simulink model "sei"  (Simulink 6.2)
settings: Solver=ode45  StartTime=0.0  StopTime=10.0  RelTol=1e-3
libraries: dsparch4 x287, cdsEpicsOut x108, cdsEpicsIn x18, cdsRms x18, Matrix8x x15, cdsSwitch1 x12, cdsProduct x9, Matrix88 x9, cdsSwitch x6, cdsSubtract8 x3, cdsRampSwitch x3, cdsSWD1 x3
(part 3 of 6)

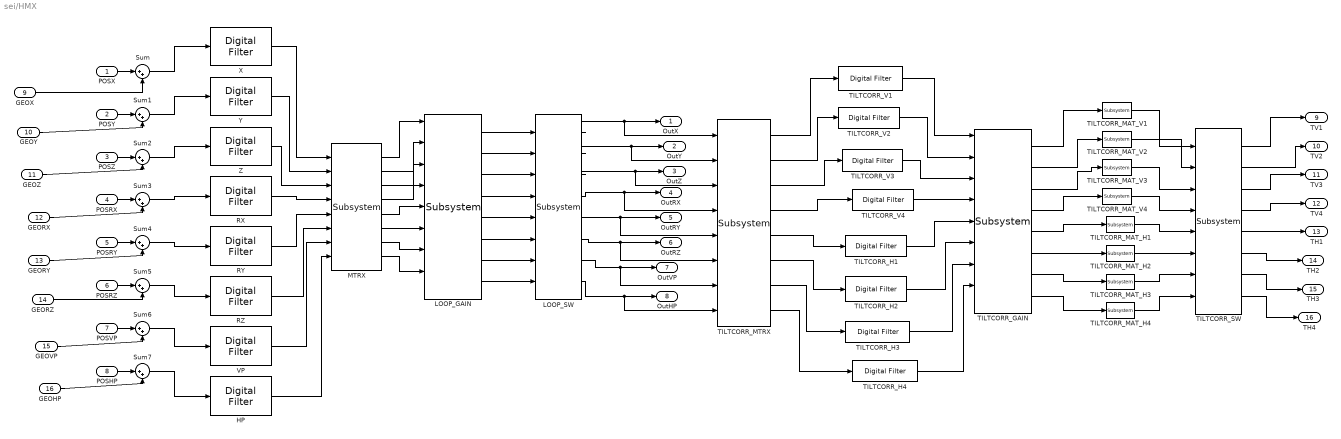
== system sei/HMX ==
  POSX : Inport  Port=1  LatchInput=off
  POSY : Inport  Port=2  LatchInput=off
  POSZ : Inport  Port=3  LatchInput=off
  POSRX : Inport  Port=4  LatchInput=off
  POSRY : Inport  Port=5  LatchInput=off
  POSRZ : Inport  Port=6  LatchInput=off
  POSVP : Inport  Port=7  LatchInput=off
  POSHP : Inport  Port=8  LatchInput=off
  GEOX : Inport  Port=9  LatchInput=off
  GEOY : Inport  Port=10  LatchInput=off
  GEOZ : Inport  Port=11  LatchInput=off
  GEORX : Inport  Port=12  LatchInput=off
  GEORY : Inport  Port=13  LatchInput=off
  GEORZ : Inport  Port=14  LatchInput=off
  GEOVP : Inport  Port=15  LatchInput=off
  GEOHP : Inport  Port=16  LatchInput=off
  HP : dsparch4/Digital Filter  DialogController=dspDDGCreate  DialogControllerArgs=DataTag93  TypePopup=IIR (poles & zeros)  IIRFiltStruct=Direct form II transposed  AllPoleFiltStruct=Direct form  FIRFiltStruct=Direct form  CoeffSource=Specify via dialog  NumCoeffs=[1 2]  DenCoeffs=[1 0.1]  BiQuadCoeffs=[1 0.3 0.4 1 0.1 0.2]  LatticeCoeffs=[0.2 0.4]  denIgnore=on  FiltPerSampPopup=One filter per frame  IC=0  ICnum=0  ICden=0  roundingMode=Floor  overflowMode=off  ScaleValues=1  scaleValueFracLength=14  stageInFracLength=15  stageOutFracLength=15
  LOOP_GAIN : cdsProduct/Subsystem
      settings: AttributesFormatString=%<ReferenceBlock>
  LOOP_SW : cdsSwitch1/Subsystem
      settings: AttributesFormatString=%<ReferenceBlock>
  MTRX : Matrix8x/Subsystem
  RX : dsparch4/Digital Filter  DialogController=dspDDGCreate  DialogControllerArgs=DataTag94  TypePopup=IIR (poles & zeros)  IIRFiltStruct=Direct form II transposed  AllPoleFiltStruct=Direct form  FIRFiltStruct=Direct form  CoeffSource=Specify via dialog  NumCoeffs=[1 2]  DenCoeffs=[1 0.1]  BiQuadCoeffs=[1 0.3 0.4 1 0.1 0.2]  LatticeCoeffs=[0.2 0.4]  denIgnore=on  FiltPerSampPopup=One filter per frame  IC=0  ICnum=0  ICden=0  roundingMode=Floor  overflowMode=off  ScaleValues=1  scaleValueFracLength=14  stageInFracLength=15  stageOutFracLength=15
  RY : dsparch4/Digital Filter  DialogController=dspDDGCreate  DialogControllerArgs=DataTag95  TypePopup=IIR (poles & zeros)  IIRFiltStruct=Direct form II transposed  AllPoleFiltStruct=Direct form  FIRFiltStruct=Direct form  CoeffSource=Specify via dialog  NumCoeffs=[1 2]  DenCoeffs=[1 0.1]  BiQuadCoeffs=[1 0.3 0.4 1 0.1 0.2]  LatticeCoeffs=[0.2 0.4]  denIgnore=on  FiltPerSampPopup=One filter per frame  IC=0  ICnum=0  ICden=0  roundingMode=Floor  overflowMode=off  ScaleValues=1  scaleValueFracLength=14  stageInFracLength=15  stageOutFracLength=15
  RZ : dsparch4/Digital Filter  DialogController=dspDDGCreate  DialogControllerArgs=DataTag96  TypePopup=IIR (poles & zeros)  IIRFiltStruct=Direct form II transposed  AllPoleFiltStruct=Direct form  FIRFiltStruct=Direct form  CoeffSource=Specify via dialog  NumCoeffs=[1 2]  DenCoeffs=[1 0.1]  BiQuadCoeffs=[1 0.3 0.4 1 0.1 0.2]  LatticeCoeffs=[0.2 0.4]  denIgnore=on  FiltPerSampPopup=One filter per frame  IC=0  ICnum=0  ICden=0  roundingMode=Floor  overflowMode=off  ScaleValues=1  scaleValueFracLength=14  stageInFracLength=15  stageOutFracLength=15
  Sum{,1..7} (8 alike) : Sum  Inputs=|++
  TILTCORR_GAIN : cdsProduct/Subsystem
      settings: AttributesFormatString=%<ReferenceBlock>
  TILTCORR_H1 : dsparch4/Digital Filter  DialogController=dspDDGCreate  DialogControllerArgs=DataTag97  TypePopup=IIR (poles & zeros)  IIRFiltStruct=Direct form II transposed  AllPoleFiltStruct=Direct form  FIRFiltStruct=Direct form  CoeffSource=Specify via dialog  NumCoeffs=[1 2]  DenCoeffs=[1 0.1]  BiQuadCoeffs=[1 0.3 0.4 1 0.1 0.2]  LatticeCoeffs=[0.2 0.4]  denIgnore=on  FiltPerSampPopup=One filter per frame  IC=0  ICnum=0  ICden=0  roundingMode=Floor  overflowMode=off  ScaleValues=1  scaleValueFracLength=14  stageInFracLength=15  stageOutFracLength=15
  TILTCORR_H2 : dsparch4/Digital Filter  DialogController=dspDDGCreate  DialogControllerArgs=DataTag98  TypePopup=IIR (poles & zeros)  IIRFiltStruct=Direct form II transposed  AllPoleFiltStruct=Direct form  FIRFiltStruct=Direct form  CoeffSource=Specify via dialog  NumCoeffs=[1 2]  DenCoeffs=[1 0.1]  BiQuadCoeffs=[1 0.3 0.4 1 0.1 0.2]  LatticeCoeffs=[0.2 0.4]  denIgnore=on  FiltPerSampPopup=One filter per frame  IC=0  ICnum=0  ICden=0  roundingMode=Floor  overflowMode=off  ScaleValues=1  scaleValueFracLength=14  stageInFracLength=15  stageOutFracLength=15
  TILTCORR_H3 : dsparch4/Digital Filter  DialogController=dspDDGCreate  DialogControllerArgs=DataTag99  TypePopup=IIR (poles & zeros)  IIRFiltStruct=Direct form II transposed  AllPoleFiltStruct=Direct form  FIRFiltStruct=Direct form  CoeffSource=Specify via dialog  NumCoeffs=[1 2]  DenCoeffs=[1 0.1]  BiQuadCoeffs=[1 0.3 0.4 1 0.1 0.2]  LatticeCoeffs=[0.2 0.4]  denIgnore=on  FiltPerSampPopup=One filter per frame  IC=0  ICnum=0  ICden=0  roundingMode=Floor  overflowMode=off  ScaleValues=1  scaleValueFracLength=14  stageInFracLength=15  stageOutFracLength=15
  TILTCORR_H4 : dsparch4/Digital Filter  DialogController=dspDDGCreate  DialogControllerArgs=DataTag100  TypePopup=IIR (poles & zeros)  IIRFiltStruct=Direct form II transposed  AllPoleFiltStruct=Direct form  FIRFiltStruct=Direct form  CoeffSource=Specify via dialog  NumCoeffs=[1 2]  DenCoeffs=[1 0.1]  BiQuadCoeffs=[1 0.3 0.4 1 0.1 0.2]  LatticeCoeffs=[0.2 0.4]  denIgnore=on  FiltPerSampPopup=One filter per frame  IC=0  ICnum=0  ICden=0  roundingMode=Floor  overflowMode=off  ScaleValues=1  scaleValueFracLength=14  stageInFracLength=15  stageOutFracLength=15
  TILTCORR_MAT_H{1..4} (4 alike) : cdsEpicsOut/Subsystem
  TILTCORR_MAT_V{1..4} (4 alike) : cdsEpicsOut/Subsystem
  TILTCORR_MTRX : Matrix8x/Subsystem
  TILTCORR_SW : cdsSwitch1/Subsystem
      settings: AttributesFormatString=%<ReferenceBlock>
  TILTCORR_V1 : dsparch4/Digital Filter  DialogController=dspDDGCreate  DialogControllerArgs=DataTag101  TypePopup=IIR (poles & zeros)  IIRFiltStruct=Direct form II transposed  AllPoleFiltStruct=Direct form  FIRFiltStruct=Direct form  CoeffSource=Specify via dialog  NumCoeffs=[1 2]  DenCoeffs=[1 0.1]  BiQuadCoeffs=[1 0.3 0.4 1 0.1 0.2]  LatticeCoeffs=[0.2 0.4]  denIgnore=on  FiltPerSampPopup=One filter per frame  IC=0  ICnum=0  ICden=0  roundingMode=Floor  overflowMode=off  ScaleValues=1  scaleValueFracLength=14  stageInFracLength=15  stageOutFracLength=15
  TILTCORR_V2 : dsparch4/Digital Filter  DialogController=dspDDGCreate  DialogControllerArgs=DataTag102  TypePopup=IIR (poles & zeros)  IIRFiltStruct=Direct form II transposed  AllPoleFiltStruct=Direct form  FIRFiltStruct=Direct form  CoeffSource=Specify via dialog  NumCoeffs=[1 2]  DenCoeffs=[1 0.1]  BiQuadCoeffs=[1 0.3 0.4 1 0.1 0.2]  LatticeCoeffs=[0.2 0.4]  denIgnore=on  FiltPerSampPopup=One filter per frame  IC=0  ICnum=0  ICden=0  roundingMode=Floor  overflowMode=off  ScaleValues=1  scaleValueFracLength=14  stageInFracLength=15  stageOutFracLength=15
  TILTCORR_V3 : dsparch4/Digital Filter  DialogController=dspDDGCreate  DialogControllerArgs=DataTag103  TypePopup=IIR (poles & zeros)  IIRFiltStruct=Direct form II transposed  AllPoleFiltStruct=Direct form  FIRFiltStruct=Direct form  CoeffSource=Specify via dialog  NumCoeffs=[1 2]  DenCoeffs=[1 0.1]  BiQuadCoeffs=[1 0.3 0.4 1 0.1 0.2]  LatticeCoeffs=[0.2 0.4]  denIgnore=on  FiltPerSampPopup=One filter per frame  IC=0  ICnum=0  ICden=0  roundingMode=Floor  overflowMode=off  ScaleValues=1  scaleValueFracLength=14  stageInFracLength=15  stageOutFracLength=15
  TILTCORR_V4 : dsparch4/Digital Filter  DialogController=dspDDGCreate  DialogControllerArgs=DataTag104  TypePopup=IIR (poles & zeros)  IIRFiltStruct=Direct form II transposed  AllPoleFiltStruct=Direct form  FIRFiltStruct=Direct form  CoeffSource=Specify via dialog  NumCoeffs=[1 2]  DenCoeffs=[1 0.1]  BiQuadCoeffs=[1 0.3 0.4 1 0.1 0.2]  LatticeCoeffs=[0.2 0.4]  denIgnore=on  FiltPerSampPopup=One filter per frame  IC=0  ICnum=0  ICden=0  roundingMode=Floor  overflowMode=off  ScaleValues=1  scaleValueFracLength=14  stageInFracLength=15  stageOutFracLength=15
  VP : dsparch4/Digital Filter  DialogController=dspDDGCreate  DialogControllerArgs=DataTag105  TypePopup=IIR (poles & zeros)  IIRFiltStruct=Direct form II transposed  AllPoleFiltStruct=Direct form  FIRFiltStruct=Direct form  CoeffSource=Specify via dialog  NumCoeffs=[1 2]  DenCoeffs=[1 0.1]  BiQuadCoeffs=[1 0.3 0.4 1 0.1 0.2]  LatticeCoeffs=[0.2 0.4]  denIgnore=on  FiltPerSampPopup=One filter per frame  IC=0  ICnum=0  ICden=0  roundingMode=Floor  overflowMode=off  ScaleValues=1  scaleValueFracLength=14  stageInFracLength=15  stageOutFracLength=15
  X : dsparch4/Digital Filter  DialogController=dspDDGCreate  DialogControllerArgs=DataTag106  TypePopup=IIR (poles & zeros)  IIRFiltStruct=Direct form II transposed  AllPoleFiltStruct=Direct form  FIRFiltStruct=Direct form  CoeffSource=Specify via dialog  NumCoeffs=[1 2]  DenCoeffs=[1 0.1]  BiQuadCoeffs=[1 0.3 0.4 1 0.1 0.2]  LatticeCoeffs=[0.2 0.4]  denIgnore=on  FiltPerSampPopup=One filter per frame  IC=0  ICnum=0  ICden=0  roundingMode=Floor  overflowMode=off  ScaleValues=1  scaleValueFracLength=14  stageInFracLength=15  stageOutFracLength=15
  Y : dsparch4/Digital Filter  DialogController=dspDDGCreate  DialogControllerArgs=DataTag107  TypePopup=IIR (poles & zeros)  IIRFiltStruct=Direct form II transposed  AllPoleFiltStruct=Direct form  FIRFiltStruct=Direct form  CoeffSource=Specify via dialog  NumCoeffs=[1 2]  DenCoeffs=[1 0.1]  BiQuadCoeffs=[1 0.3 0.4 1 0.1 0.2]  LatticeCoeffs=[0.2 0.4]  denIgnore=on  FiltPerSampPopup=One filter per frame  IC=0  ICnum=0  ICden=0  roundingMode=Floor  overflowMode=off  ScaleValues=1  scaleValueFracLength=14  stageInFracLength=15  stageOutFracLength=15
  Z : dsparch4/Digital Filter  DialogController=dspDDGCreate  DialogControllerArgs=DataTag108  TypePopup=IIR (poles & zeros)  IIRFiltStruct=Direct form II transposed  AllPoleFiltStruct=Direct form  FIRFiltStruct=Direct form  CoeffSource=Specify via dialog  NumCoeffs=[1 2]  DenCoeffs=[1 0.1]  BiQuadCoeffs=[1 0.3 0.4 1 0.1 0.2]  LatticeCoeffs=[0.2 0.4]  denIgnore=on  FiltPerSampPopup=One filter per frame  IC=0  ICnum=0  ICden=0  roundingMode=Floor  overflowMode=off  ScaleValues=1  scaleValueFracLength=14  stageInFracLength=15  stageOutFracLength=15
  OutX : Outport
  OutY : Outport  Port=2
  OutZ : Outport  Port=3
  OutRX : Outport  Port=4
  OutRY : Outport  Port=5
  OutRZ : Outport  Port=6
  OutVP : Outport  Port=7
  OutHP : Outport  Port=8
  TV1 : Outport  Port=9
  TV2 : Outport  Port=10
  TV3 : Outport  Port=11
  TV4 : Outport  Port=12
  TH1 : Outport  Port=13
  TH2 : Outport  Port=14
  TH3 : Outport  Port=15
  TH4 : Outport  Port=16
  wires:
  Sum/1 -> X/1
  Sum1/1 -> Y/1
  Sum2/1 -> Z/1
  Sum3/1 -> RX/1
  Sum4/1 -> RY/1
  Sum5/1 -> RZ/1
  Sum6/1 -> VP/1
  Sum7/1 -> HP/1
  X/1 -> MTRX/1
  Y/1 -> MTRX/2
  Z/1 -> MTRX/3
  RX/1 -> MTRX/4
  RY/1 -> MTRX/5
  RZ/1 -> MTRX/6
  VP/1 -> MTRX/7
  HP/1 -> MTRX/8
  POSX/1 -> Sum/1
  GEOX/1 -> Sum/2
  POSY/1 -> Sum1/1
  GEOY/1 -> Sum1/2
  POSZ/1 -> Sum2/1
  GEOZ/1 -> Sum2/2
  POSRX/1 -> Sum3/1
  GEORX/1 -> Sum3/2
  POSRY/1 -> Sum4/1
  GEORY/1 -> Sum4/2
  POSRZ/1 -> Sum5/1
  GEORZ/1 -> Sum5/2
  POSVP/1 -> Sum6/1
  GEOVP/1 -> Sum6/2
  POSHP/1 -> Sum7/1
  GEOHP/1 -> Sum7/2
  LOOP_GAIN/1 -> LOOP_SW/1
  LOOP_GAIN/2 -> LOOP_SW/2
  LOOP_GAIN/3 -> LOOP_SW/3
  LOOP_GAIN/4 -> LOOP_SW/4
  LOOP_GAIN/5 -> LOOP_SW/5
  LOOP_GAIN/6 -> LOOP_SW/6
  LOOP_GAIN/7 -> LOOP_SW/7
  LOOP_GAIN/8 -> LOOP_SW/8
  LOOP_SW/1 -> OutX/1, TILTCORR_MTRX/1
  LOOP_SW/2 -> OutY/1, TILTCORR_MTRX/2
  LOOP_SW/3 -> OutZ/1, TILTCORR_MTRX/3
  LOOP_SW/4 -> OutRX/1, TILTCORR_MTRX/4
  LOOP_SW/5 -> OutRY/1, TILTCORR_MTRX/5
  LOOP_SW/6 -> OutRZ/1, TILTCORR_MTRX/6
  LOOP_SW/7 -> OutVP/1, TILTCORR_MTRX/7
  LOOP_SW/8 -> OutHP/1, TILTCORR_MTRX/8
  MTRX/1 -> LOOP_GAIN/1
  MTRX/2 -> LOOP_GAIN/2
  MTRX/3 -> LOOP_GAIN/3
  MTRX/4 -> LOOP_GAIN/4
  MTRX/5 -> LOOP_GAIN/5
  MTRX/6 -> LOOP_GAIN/6
  MTRX/7 -> LOOP_GAIN/7
  MTRX/8 -> LOOP_GAIN/8
  TILTCORR_MTRX/1 -> TILTCORR_V1/1
  TILTCORR_MTRX/2 -> TILTCORR_V2/1
  TILTCORR_MTRX/3 -> TILTCORR_V3/1
  TILTCORR_MTRX/4 -> TILTCORR_V4/1
  TILTCORR_MTRX/5 -> TILTCORR_H1/1
  TILTCORR_MTRX/6 -> TILTCORR_H2/1
  TILTCORR_MTRX/7 -> TILTCORR_H3/1
  TILTCORR_MTRX/8 -> TILTCORR_H4/1
  TILTCORR_V1/1 -> TILTCORR_GAIN/1
  TILTCORR_V2/1 -> TILTCORR_GAIN/2
  TILTCORR_V3/1 -> TILTCORR_GAIN/3
  TILTCORR_V4/1 -> TILTCORR_GAIN/4
  TILTCORR_H1/1 -> TILTCORR_GAIN/5
  TILTCORR_H2/1 -> TILTCORR_GAIN/6
  TILTCORR_H3/1 -> TILTCORR_GAIN/7
  TILTCORR_H4/1 -> TILTCORR_GAIN/8
  TILTCORR_GAIN/1 -> TILTCORR_MAT_V1/1
  TILTCORR_GAIN/2 -> TILTCORR_MAT_V2/1
  TILTCORR_GAIN/3 -> TILTCORR_MAT_V3/1
  TILTCORR_GAIN/4 -> TILTCORR_MAT_V4/1
  TILTCORR_GAIN/5 -> TILTCORR_MAT_H1/1
  TILTCORR_GAIN/6 -> TILTCORR_MAT_H2/1
  TILTCORR_GAIN/7 -> TILTCORR_MAT_H3/1
  TILTCORR_GAIN/8 -> TILTCORR_MAT_H4/1
  TILTCORR_MAT_V1/1 -> TILTCORR_SW/1
  TILTCORR_MAT_V2/1 -> TILTCORR_SW/2
  TILTCORR_MAT_V3/1 -> TILTCORR_SW/3
  TILTCORR_MAT_V4/1 -> TILTCORR_SW/4
  TILTCORR_MAT_H1/1 -> TILTCORR_SW/5
  TILTCORR_MAT_H2/1 -> TILTCORR_SW/6
  TILTCORR_MAT_H3/1 -> TILTCORR_SW/7
  TILTCORR_MAT_H4/1 -> TILTCORR_SW/8
  TILTCORR_SW/1 -> TV1/1
  TILTCORR_SW/2 -> TV2/1
  TILTCORR_SW/3 -> TV3/1
  TILTCORR_SW/4 -> TV4/1
  TILTCORR_SW/5 -> TH1/1
  TILTCORR_SW/6 -> TH2/1
  TILTCORR_SW/7 -> TH3/1
  TILTCORR_SW/8 -> TH4/1

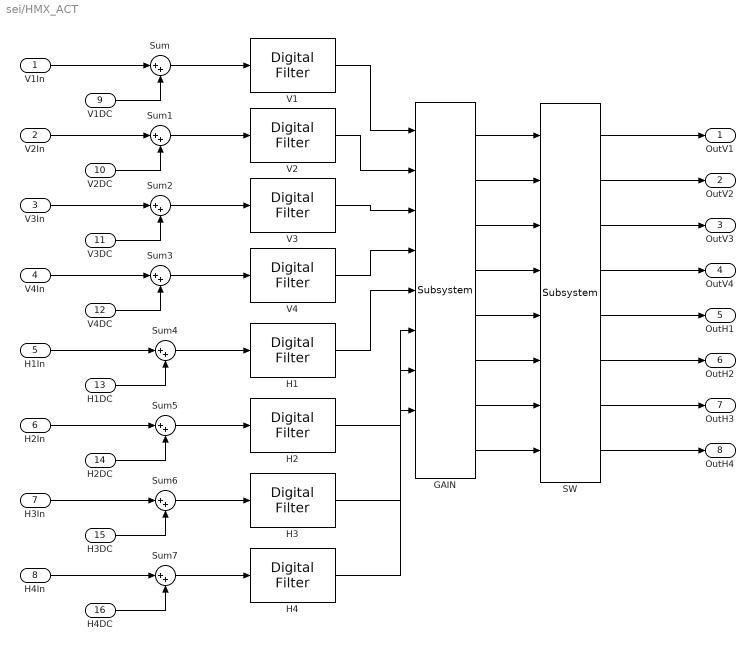
== system sei/HMX_ACT ==
  V1In : Inport  Port=1  LatchInput=off
  V2In : Inport  Port=2  LatchInput=off
  V3In : Inport  Port=3  LatchInput=off
  V4In : Inport  Port=4  LatchInput=off
  H1In : Inport  Port=5  LatchInput=off
  H2In : Inport  Port=6  LatchInput=off
  H3In : Inport  Port=7  LatchInput=off
  H4In : Inport  Port=8  LatchInput=off
  V1DC : Inport  Port=9  LatchInput=off
  V2DC : Inport  Port=10  LatchInput=off
  V3DC : Inport  Port=11  LatchInput=off
  V4DC : Inport  Port=12  LatchInput=off
  H1DC : Inport  Port=13  LatchInput=off
  H2DC : Inport  Port=14  LatchInput=off
  H3DC : Inport  Port=15  LatchInput=off
  H4DC : Inport  Port=16  LatchInput=off
  GAIN : cdsProduct/Subsystem
  H1 : dsparch4/Digital Filter  DialogController=dspDDGCreate  DialogControllerArgs=DataTag109  TypePopup=IIR (poles & zeros)  IIRFiltStruct=Direct form II transposed  AllPoleFiltStruct=Direct form  FIRFiltStruct=Direct form  CoeffSource=Specify via dialog  NumCoeffs=[1 2]  DenCoeffs=[1 0.1]  BiQuadCoeffs=[1 0.3 0.4 1 0.1 0.2]  LatticeCoeffs=[0.2 0.4]  denIgnore=on  FiltPerSampPopup=One filter per frame  IC=0  ICnum=0  ICden=0  roundingMode=Floor  overflowMode=off  ScaleValues=1  scaleValueFracLength=14  stageInFracLength=15  stageOutFracLength=15
  H2 : dsparch4/Digital Filter  DialogController=dspDDGCreate  DialogControllerArgs=DataTag110  TypePopup=IIR (poles & zeros)  IIRFiltStruct=Direct form II transposed  AllPoleFiltStruct=Direct form  FIRFiltStruct=Direct form  CoeffSource=Specify via dialog  NumCoeffs=[1 2]  DenCoeffs=[1 0.1]  BiQuadCoeffs=[1 0.3 0.4 1 0.1 0.2]  LatticeCoeffs=[0.2 0.4]  denIgnore=on  FiltPerSampPopup=One filter per frame  IC=0  ICnum=0  ICden=0  roundingMode=Floor  overflowMode=off  ScaleValues=1  scaleValueFracLength=14  stageInFracLength=15  stageOutFracLength=15
  H3 : dsparch4/Digital Filter  DialogController=dspDDGCreate  DialogControllerArgs=DataTag111  TypePopup=IIR (poles & zeros)  IIRFiltStruct=Direct form II transposed  AllPoleFiltStruct=Direct form  FIRFiltStruct=Direct form  CoeffSource=Specify via dialog  NumCoeffs=[1 2]  DenCoeffs=[1 0.1]  BiQuadCoeffs=[1 0.3 0.4 1 0.1 0.2]  LatticeCoeffs=[0.2 0.4]  denIgnore=on  FiltPerSampPopup=One filter per frame  IC=0  ICnum=0  ICden=0  roundingMode=Floor  overflowMode=off  ScaleValues=1  scaleValueFracLength=14  stageInFracLength=15  stageOutFracLength=15
  H4 : dsparch4/Digital Filter  DialogController=dspDDGCreate  DialogControllerArgs=DataTag112  TypePopup=IIR (poles & zeros)  IIRFiltStruct=Direct form II transposed  AllPoleFiltStruct=Direct form  FIRFiltStruct=Direct form  CoeffSource=Specify via dialog  NumCoeffs=[1 2]  DenCoeffs=[1 0.1]  BiQuadCoeffs=[1 0.3 0.4 1 0.1 0.2]  LatticeCoeffs=[0.2 0.4]  denIgnore=on  FiltPerSampPopup=One filter per frame  IC=0  ICnum=0  ICden=0  roundingMode=Floor  overflowMode=off  ScaleValues=1  scaleValueFracLength=14  stageInFracLength=15  stageOutFracLength=15
  SW : cdsSwitch1/Subsystem
  Sum{,1..7} (8 alike) : Sum  Inputs=|++
  V1 : dsparch4/Digital Filter  DialogController=dspDDGCreate  DialogControllerArgs=DataTag113  TypePopup=IIR (poles & zeros)  IIRFiltStruct=Direct form II transposed  AllPoleFiltStruct=Direct form  FIRFiltStruct=Direct form  CoeffSource=Specify via dialog  NumCoeffs=[1 2]  DenCoeffs=[1 0.1]  BiQuadCoeffs=[1 0.3 0.4 1 0.1 0.2]  LatticeCoeffs=[0.2 0.4]  denIgnore=on  FiltPerSampPopup=One filter per frame  IC=0  ICnum=0  ICden=0  roundingMode=Floor  overflowMode=off  ScaleValues=1  scaleValueFracLength=14  stageInFracLength=15  stageOutFracLength=15
  V2 : dsparch4/Digital Filter  DialogController=dspDDGCreate  DialogControllerArgs=DataTag114  TypePopup=IIR (poles & zeros)  IIRFiltStruct=Direct form II transposed  AllPoleFiltStruct=Direct form  FIRFiltStruct=Direct form  CoeffSource=Specify via dialog  NumCoeffs=[1 2]  DenCoeffs=[1 0.1]  BiQuadCoeffs=[1 0.3 0.4 1 0.1 0.2]  LatticeCoeffs=[0.2 0.4]  denIgnore=on  FiltPerSampPopup=One filter per frame  IC=0  ICnum=0  ICden=0  roundingMode=Floor  overflowMode=off  ScaleValues=1  scaleValueFracLength=14  stageInFracLength=15  stageOutFracLength=15
  V3 : dsparch4/Digital Filter  DialogController=dspDDGCreate  DialogControllerArgs=DataTag115  TypePopup=IIR (poles & zeros)  IIRFiltStruct=Direct form II transposed  AllPoleFiltStruct=Direct form  FIRFiltStruct=Direct form  CoeffSource=Specify via dialog  NumCoeffs=[1 2]  DenCoeffs=[1 0.1]  BiQuadCoeffs=[1 0.3 0.4 1 0.1 0.2]  LatticeCoeffs=[0.2 0.4]  denIgnore=on  FiltPerSampPopup=One filter per frame  IC=0  ICnum=0  ICden=0  roundingMode=Floor  overflowMode=off  ScaleValues=1  scaleValueFracLength=14  stageInFracLength=15  stageOutFracLength=15
  V4 : dsparch4/Digital Filter  DialogController=dspDDGCreate  DialogControllerArgs=DataTag116  TypePopup=IIR (poles & zeros)  IIRFiltStruct=Direct form II transposed  AllPoleFiltStruct=Direct form  FIRFiltStruct=Direct form  CoeffSource=Specify via dialog  NumCoeffs=[1 2]  DenCoeffs=[1 0.1]  BiQuadCoeffs=[1 0.3 0.4 1 0.1 0.2]  LatticeCoeffs=[0.2 0.4]  denIgnore=on  FiltPerSampPopup=One filter per frame  IC=0  ICnum=0  ICden=0  roundingMode=Floor  overflowMode=off  ScaleValues=1  scaleValueFracLength=14  stageInFracLength=15  stageOutFracLength=15
  OutV1 : Outport
  OutV2 : Outport  Port=2
  OutV3 : Outport  Port=3
  OutV4 : Outport  Port=4
  OutH1 : Outport  Port=5
  OutH2 : Outport  Port=6
  OutH3 : Outport  Port=7
  OutH4 : Outport  Port=8
  wires:
  GAIN/1 -> SW/1
  GAIN/2 -> SW/2
  GAIN/3 -> SW/3
  GAIN/4 -> SW/4
  GAIN/5 -> SW/5
  GAIN/6 -> SW/6
  GAIN/7 -> SW/7
  GAIN/8 -> SW/8
  V1DC/1 -> Sum/2
  V2DC/1 -> Sum1/2
  V3DC/1 -> Sum2/2
  V4DC/1 -> Sum3/2
  H1DC/1 -> Sum4/2
  H2DC/1 -> Sum5/2
  H3DC/1 -> Sum6/2
  H4DC/1 -> Sum7/2
  Sum4/1 -> H1/1
  Sum5/1 -> H2/1
  Sum6/1 -> H3/1
  Sum7/1 -> H4/1
  Sum3/1 -> V4/1
  Sum2/1 -> V3/1
  Sum1/1 -> V2/1
  Sum/1 -> V1/1
  V1In/1 -> Sum/1
  V2In/1 -> Sum1/1
  V3In/1 -> Sum2/1
  V4In/1 -> Sum3/1
  H1In/1 -> Sum4/1
  H2In/1 -> Sum5/1
  H3In/1 -> Sum6/1
  H4In/1 -> Sum7/1
  V1/1 -> GAIN/1
  V2/1 -> GAIN/2
  V3/1 -> GAIN/3
  V4/1 -> GAIN/4
  H1/1 -> GAIN/5
  H2/1 -> GAIN/6
  H3/1 -> GAIN/7
  H4/1 -> GAIN/8
  SW/1 -> OutV1/1
  SW/2 -> OutV2/1
  SW/3 -> OutV3/1
  SW/4 -> OutV4/1
  SW/5 -> OutH1/1
  SW/6 -> OutH2/1
  SW/7 -> OutH3/1
  SW/8 -> OutH4/1

== system sei/HMX_DC_BIAS ==
  {1..6} (6 alike) : cdsEpicsIn/Subsystem
  MTRX : Matrix8x/Subsystem
  SW : cdsSwitch1/Subsystem
  V1 : Outport
  V2 : Outport  Port=2
  V3 : Outport  Port=3
  V4 : Outport  Port=4
  H1 : Outport  Port=5
  H2 : Outport  Port=6
  H3 : Outport  Port=7
  H4 : Outport  Port=8
  wires:
  1/1 -> MTRX/1
  2/1 -> MTRX/2
  3/1 -> MTRX/3
  4/1 -> MTRX/4
  5/1 -> MTRX/5
  6/1 -> MTRX/6
  MTRX/1 -> SW/1
  MTRX/2 -> SW/2
  MTRX/3 -> SW/3
  MTRX/4 -> SW/4
  MTRX/5 -> SW/5
  MTRX/6 -> SW/6
  MTRX/7 -> SW/7
  MTRX/8 -> SW/8
  SW/1 -> V1/1
  SW/2 -> V2/1
  SW/3 -> V3/1
  SW/4 -> V4/1
  SW/5 -> H1/1
  SW/6 -> H2/1
  SW/7 -> H3/1
  SW/8 -> H4/1

== system sei/HMX_FIR ==
  X1 : Inport  Port=1  LatchInput=off
  Y1 : Inport  Port=2  LatchInput=off
  X2 : Inport  Port=3  LatchInput=off
  Y2 : Inport  Port=4  LatchInput=off
  MTRX : Matrix88/Subsystem
  X_OUT : dsparch4/Digital Filter  DialogController=dspDDGCreate  DialogControllerArgs=DataTag117  TypePopup=IIR (poles & zeros)  IIRFiltStruct=Direct form II transposed  AllPoleFiltStruct=Direct form  FIRFiltStruct=Direct form  CoeffSource=Specify via dialog  NumCoeffs=[1 2]  DenCoeffs=[1 0.1]  BiQuadCoeffs=[1 0.3 0.4 1 0.1 0.2]  LatticeCoeffs=[0.2 0.4]  denIgnore=on  FiltPerSampPopup=One filter per frame  IC=0  ICnum=0  ICden=0  roundingMode=Floor  overflowMode=off  ScaleValues=1  scaleValueFracLength=14  stageInFracLength=15  stageOutFracLength=15
  Y_OUT : dsparch4/Digital Filter  DialogController=dspDDGCreate  DialogControllerArgs=DataTag118  TypePopup=IIR (poles & zeros)  IIRFiltStruct=Direct form II transposed  AllPoleFiltStruct=Direct form  FIRFiltStruct=Direct form  CoeffSource=Specify via dialog  NumCoeffs=[1 2]  DenCoeffs=[1 0.1]  BiQuadCoeffs=[1 0.3 0.4 1 0.1 0.2]  LatticeCoeffs=[0.2 0.4]  denIgnore=on  FiltPerSampPopup=One filter per frame  IC=0  ICnum=0  ICden=0  roundingMode=Floor  overflowMode=off  ScaleValues=1  scaleValueFracLength=14  stageInFracLength=15  stageOutFracLength=15
  X : Outport
  Y : Outport  Port=2
  wires:
  MTRX/1 -> X_OUT/1
  MTRX/2 -> Y_OUT/1
  X1/1 -> MTRX/1
  X_OUT/1 -> X/1
  Y1/1 -> MTRX/2
  X2/1 -> MTRX/3
  Y2/1 -> MTRX/4
  Y_OUT/1 -> Y/1

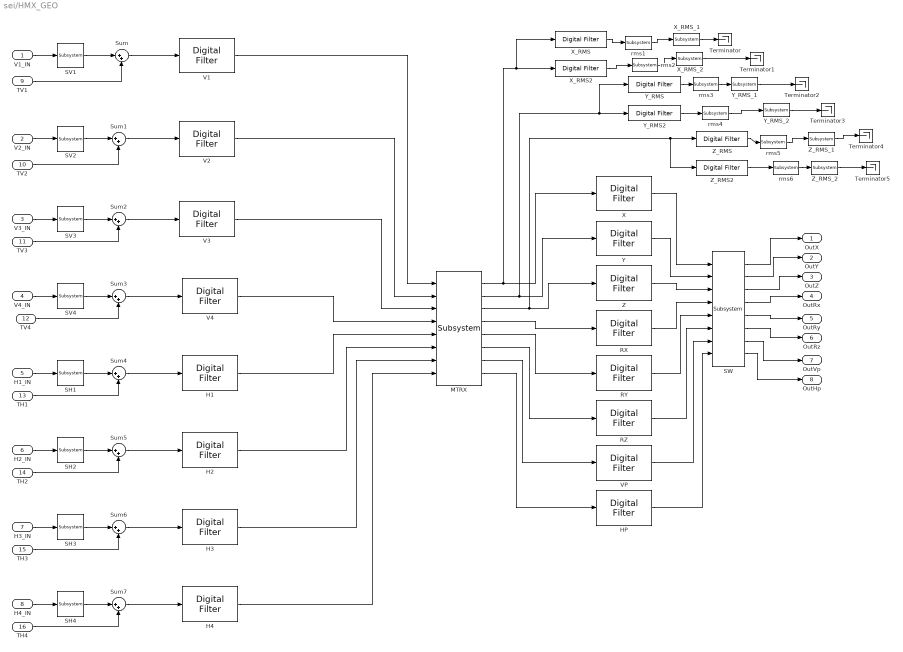
== system sei/HMX_GEO ==
  V1_IN : Inport  Port=1  LatchInput=off
  V2_IN : Inport  Port=2  LatchInput=off
  V3_IN : Inport  Port=3  LatchInput=off
  V4_IN : Inport  Port=4  LatchInput=off
  H1_IN : Inport  Port=5  LatchInput=off
  H2_IN : Inport  Port=6  LatchInput=off
  H3_IN : Inport  Port=7  LatchInput=off
  H4_IN : Inport  Port=8  LatchInput=off
  TV1 : Inport  Port=9  LatchInput=off
  TV2 : Inport  Port=10  LatchInput=off
  TV3 : Inport  Port=11  LatchInput=off
  TV4 : Inport  Port=12  LatchInput=off
  TH1 : Inport  Port=13  LatchInput=off
  TH2 : Inport  Port=14  LatchInput=off
  TH3 : Inport  Port=15  LatchInput=off
  TH4 : Inport  Port=16  LatchInput=off
  H1 : dsparch4/Digital Filter  DialogController=dspDDGCreate  DialogControllerArgs=DataTag119  TypePopup=IIR (poles & zeros)  IIRFiltStruct=Direct form II transposed  AllPoleFiltStruct=Direct form  FIRFiltStruct=Direct form  CoeffSource=Specify via dialog  NumCoeffs=[1 2]  DenCoeffs=[1 0.1]  BiQuadCoeffs=[1 0.3 0.4 1 0.1 0.2]  LatticeCoeffs=[0.2 0.4]  denIgnore=on  FiltPerSampPopup=One filter per frame  IC=0  ICnum=0  ICden=0  roundingMode=Floor  overflowMode=off  ScaleValues=1  scaleValueFracLength=14  stageInFracLength=15  stageOutFracLength=15
  H2 : dsparch4/Digital Filter  DialogController=dspDDGCreate  DialogControllerArgs=DataTag120  TypePopup=IIR (poles & zeros)  IIRFiltStruct=Direct form II transposed  AllPoleFiltStruct=Direct form  FIRFiltStruct=Direct form  CoeffSource=Specify via dialog  NumCoeffs=[1 2]  DenCoeffs=[1 0.1]  BiQuadCoeffs=[1 0.3 0.4 1 0.1 0.2]  LatticeCoeffs=[0.2 0.4]  denIgnore=on  FiltPerSampPopup=One filter per frame  IC=0  ICnum=0  ICden=0  roundingMode=Floor  overflowMode=off  ScaleValues=1  scaleValueFracLength=14  stageInFracLength=15  stageOutFracLength=15
  H3 : dsparch4/Digital Filter  DialogController=dspDDGCreate  DialogControllerArgs=DataTag121  TypePopup=IIR (poles & zeros)  IIRFiltStruct=Direct form II transposed  AllPoleFiltStruct=Direct form  FIRFiltStruct=Direct form  CoeffSource=Specify via dialog  NumCoeffs=[1 2]  DenCoeffs=[1 0.1]  BiQuadCoeffs=[1 0.3 0.4 1 0.1 0.2]  LatticeCoeffs=[0.2 0.4]  denIgnore=on  FiltPerSampPopup=One filter per frame  IC=0  ICnum=0  ICden=0  roundingMode=Floor  overflowMode=off  ScaleValues=1  scaleValueFracLength=14  stageInFracLength=15  stageOutFracLength=15
  H4 : dsparch4/Digital Filter  DialogController=dspDDGCreate  DialogControllerArgs=DataTag122  TypePopup=IIR (poles & zeros)  IIRFiltStruct=Direct form II transposed  AllPoleFiltStruct=Direct form  FIRFiltStruct=Direct form  CoeffSource=Specify via dialog  NumCoeffs=[1 2]  DenCoeffs=[1 0.1]  BiQuadCoeffs=[1 0.3 0.4 1 0.1 0.2]  LatticeCoeffs=[0.2 0.4]  denIgnore=on  FiltPerSampPopup=One filter per frame  IC=0  ICnum=0  ICden=0  roundingMode=Floor  overflowMode=off  ScaleValues=1  scaleValueFracLength=14  stageInFracLength=15  stageOutFracLength=15
  HP : dsparch4/Digital Filter  DialogController=dspDDGCreate  DialogControllerArgs=DataTag123  TypePopup=IIR (poles & zeros)  IIRFiltStruct=Direct form II transposed  AllPoleFiltStruct=Direct form  FIRFiltStruct=Direct form  CoeffSource=Specify via dialog  NumCoeffs=[1 2]  DenCoeffs=[1 0.1]  BiQuadCoeffs=[1 0.3 0.4 1 0.1 0.2]  LatticeCoeffs=[0.2 0.4]  denIgnore=on  FiltPerSampPopup=One filter per frame  IC=0  ICnum=0  ICden=0  roundingMode=Floor  overflowMode=off  ScaleValues=1  scaleValueFracLength=14  stageInFracLength=15  stageOutFracLength=15
  MTRX : Matrix8x/Subsystem
  RX : dsparch4/Digital Filter  DialogController=dspDDGCreate  DialogControllerArgs=DataTag124  TypePopup=IIR (poles & zeros)  IIRFiltStruct=Direct form II transposed  AllPoleFiltStruct=Direct form  FIRFiltStruct=Direct form  CoeffSource=Specify via dialog  NumCoeffs=[1 2]  DenCoeffs=[1 0.1]  BiQuadCoeffs=[1 0.3 0.4 1 0.1 0.2]  LatticeCoeffs=[0.2 0.4]  denIgnore=on  FiltPerSampPopup=One filter per frame  IC=0  ICnum=0  ICden=0  roundingMode=Floor  overflowMode=off  ScaleValues=1  scaleValueFracLength=14  stageInFracLength=15  stageOutFracLength=15
  RY : dsparch4/Digital Filter  DialogController=dspDDGCreate  DialogControllerArgs=DataTag125  TypePopup=IIR (poles & zeros)  IIRFiltStruct=Direct form II transposed  AllPoleFiltStruct=Direct form  FIRFiltStruct=Direct form  CoeffSource=Specify via dialog  NumCoeffs=[1 2]  DenCoeffs=[1 0.1]  BiQuadCoeffs=[1 0.3 0.4 1 0.1 0.2]  LatticeCoeffs=[0.2 0.4]  denIgnore=on  FiltPerSampPopup=One filter per frame  IC=0  ICnum=0  ICden=0  roundingMode=Floor  overflowMode=off  ScaleValues=1  scaleValueFracLength=14  stageInFracLength=15  stageOutFracLength=15
  RZ : dsparch4/Digital Filter  DialogController=dspDDGCreate  DialogControllerArgs=DataTag126  TypePopup=IIR (poles & zeros)  IIRFiltStruct=Direct form II transposed  AllPoleFiltStruct=Direct form  FIRFiltStruct=Direct form  CoeffSource=Specify via dialog  NumCoeffs=[1 2]  DenCoeffs=[1 0.1]  BiQuadCoeffs=[1 0.3 0.4 1 0.1 0.2]  LatticeCoeffs=[0.2 0.4]  denIgnore=on  FiltPerSampPopup=One filter per frame  IC=0  ICnum=0  ICden=0  roundingMode=Floor  overflowMode=off  ScaleValues=1  scaleValueFracLength=14  stageInFracLength=15  stageOutFracLength=15
  SH{1..4} (4 alike) : cdsEpicsOut/Subsystem
  SV{1..4} (4 alike) : cdsEpicsOut/Subsystem
  SW : cdsSwitch/Subsystem
  Sum{,1..7} (8 alike) : Sum  Inputs=|++
  Terminator{,1..5} (6 alike) : Terminator
  V1 : dsparch4/Digital Filter  DialogController=dspDDGCreate  DialogControllerArgs=DataTag127  TypePopup=IIR (poles & zeros)  IIRFiltStruct=Direct form II transposed  AllPoleFiltStruct=Direct form  FIRFiltStruct=Direct form  CoeffSource=Specify via dialog  NumCoeffs=[1 2]  DenCoeffs=[1 0.1]  BiQuadCoeffs=[1 0.3 0.4 1 0.1 0.2]  LatticeCoeffs=[0.2 0.4]  denIgnore=on  FiltPerSampPopup=One filter per frame  IC=0  ICnum=0  ICden=0  roundingMode=Floor  overflowMode=off  ScaleValues=1  scaleValueFracLength=14  stageInFracLength=15  stageOutFracLength=15
  V2 : dsparch4/Digital Filter  DialogController=dspDDGCreate  DialogControllerArgs=DataTag128  TypePopup=IIR (poles & zeros)  IIRFiltStruct=Direct form II transposed  AllPoleFiltStruct=Direct form  FIRFiltStruct=Direct form  CoeffSource=Specify via dialog  NumCoeffs=[1 2]  DenCoeffs=[1 0.1]  BiQuadCoeffs=[1 0.3 0.4 1 0.1 0.2]  LatticeCoeffs=[0.2 0.4]  denIgnore=on  FiltPerSampPopup=One filter per frame  IC=0  ICnum=0  ICden=0  roundingMode=Floor  overflowMode=off  ScaleValues=1  scaleValueFracLength=14  stageInFracLength=15  stageOutFracLength=15
  V3 : dsparch4/Digital Filter  DialogController=dspDDGCreate  DialogControllerArgs=DataTag129  TypePopup=IIR (poles & zeros)  IIRFiltStruct=Direct form II transposed  AllPoleFiltStruct=Direct form  FIRFiltStruct=Direct form  CoeffSource=Specify via dialog  NumCoeffs=[1 2]  DenCoeffs=[1 0.1]  BiQuadCoeffs=[1 0.3 0.4 1 0.1 0.2]  LatticeCoeffs=[0.2 0.4]  denIgnore=on  FiltPerSampPopup=One filter per frame  IC=0  ICnum=0  ICden=0  roundingMode=Floor  overflowMode=off  ScaleValues=1  scaleValueFracLength=14  stageInFracLength=15  stageOutFracLength=15
  V4 : dsparch4/Digital Filter  DialogController=dspDDGCreate  DialogControllerArgs=DataTag130  TypePopup=IIR (poles & zeros)  IIRFiltStruct=Direct form II transposed  AllPoleFiltStruct=Direct form  FIRFiltStruct=Direct form  CoeffSource=Specify via dialog  NumCoeffs=[1 2]  DenCoeffs=[1 0.1]  BiQuadCoeffs=[1 0.3 0.4 1 0.1 0.2]  LatticeCoeffs=[0.2 0.4]  denIgnore=on  FiltPerSampPopup=One filter per frame  IC=0  ICnum=0  ICden=0  roundingMode=Floor  overflowMode=off  ScaleValues=1  scaleValueFracLength=14  stageInFracLength=15  stageOutFracLength=15
  VP : dsparch4/Digital Filter  DialogController=dspDDGCreate  DialogControllerArgs=DataTag131  TypePopup=IIR (poles & zeros)  IIRFiltStruct=Direct form II transposed  AllPoleFiltStruct=Direct form  FIRFiltStruct=Direct form  CoeffSource=Specify via dialog  NumCoeffs=[1 2]  DenCoeffs=[1 0.1]  BiQuadCoeffs=[1 0.3 0.4 1 0.1 0.2]  LatticeCoeffs=[0.2 0.4]  denIgnore=on  FiltPerSampPopup=One filter per frame  IC=0  ICnum=0  ICden=0  roundingMode=Floor  overflowMode=off  ScaleValues=1  scaleValueFracLength=14  stageInFracLength=15  stageOutFracLength=15
  X : dsparch4/Digital Filter  DialogController=dspDDGCreate  DialogControllerArgs=DataTag132  TypePopup=IIR (poles & zeros)  IIRFiltStruct=Direct form II transposed  AllPoleFiltStruct=Direct form  FIRFiltStruct=Direct form  CoeffSource=Specify via dialog  NumCoeffs=[1 2]  DenCoeffs=[1 0.1]  BiQuadCoeffs=[1 0.3 0.4 1 0.1 0.2]  LatticeCoeffs=[0.2 0.4]  denIgnore=on  FiltPerSampPopup=One filter per frame  IC=0  ICnum=0  ICden=0  roundingMode=Floor  overflowMode=off  ScaleValues=1  scaleValueFracLength=14  stageInFracLength=15  stageOutFracLength=15
  X_RMS : dsparch4/Digital Filter  DialogController=dspDDGCreate  DialogControllerArgs=DataTag133  TypePopup=IIR (poles & zeros)  IIRFiltStruct=Direct form II transposed  AllPoleFiltStruct=Direct form  FIRFiltStruct=Direct form  CoeffSource=Specify via dialog  NumCoeffs=[1 2]  DenCoeffs=[1 0.1]  BiQuadCoeffs=[1 0.3 0.4 1 0.1 0.2]  LatticeCoeffs=[0.2 0.4]  denIgnore=on  FiltPerSampPopup=One filter per frame  IC=0  ICnum=0  ICden=0  roundingMode=Floor  overflowMode=off  ScaleValues=1  scaleValueFracLength=14  stageInFracLength=15  stageOutFracLength=15
  X_RMS2 : dsparch4/Digital Filter  DialogController=dspDDGCreate  DialogControllerArgs=DataTag134  TypePopup=IIR (poles & zeros)  IIRFiltStruct=Direct form II transposed  AllPoleFiltStruct=Direct form  FIRFiltStruct=Direct form  CoeffSource=Specify via dialog  NumCoeffs=[1 2]  DenCoeffs=[1 0.1]  BiQuadCoeffs=[1 0.3 0.4 1 0.1 0.2]  LatticeCoeffs=[0.2 0.4]  denIgnore=on  FiltPerSampPopup=One filter per frame  IC=0  ICnum=0  ICden=0  roundingMode=Floor  overflowMode=off  ScaleValues=1  scaleValueFracLength=14  stageInFracLength=15  stageOutFracLength=15
  X_RMS_1 : cdsEpicsOut/Subsystem
  X_RMS_2 : cdsEpicsOut/Subsystem
  Y : dsparch4/Digital Filter  DialogController=dspDDGCreate  DialogControllerArgs=DataTag135  TypePopup=IIR (poles & zeros)  IIRFiltStruct=Direct form II transposed  AllPoleFiltStruct=Direct form  FIRFiltStruct=Direct form  CoeffSource=Specify via dialog  NumCoeffs=[1 2]  DenCoeffs=[1 0.1]  BiQuadCoeffs=[1 0.3 0.4 1 0.1 0.2]  LatticeCoeffs=[0.2 0.4]  denIgnore=on  FiltPerSampPopup=One filter per frame  IC=0  ICnum=0  ICden=0  roundingMode=Floor  overflowMode=off  ScaleValues=1  scaleValueFracLength=14  stageInFracLength=15  stageOutFracLength=15
  Y_RMS : dsparch4/Digital Filter  DialogController=dspDDGCreate  DialogControllerArgs=DataTag136  TypePopup=IIR (poles & zeros)  IIRFiltStruct=Direct form II transposed  AllPoleFiltStruct=Direct form  FIRFiltStruct=Direct form  CoeffSource=Specify via dialog  NumCoeffs=[1 2]  DenCoeffs=[1 0.1]  BiQuadCoeffs=[1 0.3 0.4 1 0.1 0.2]  LatticeCoeffs=[0.2 0.4]  denIgnore=on  FiltPerSampPopup=One filter per frame  IC=0  ICnum=0  ICden=0  roundingMode=Floor  overflowMode=off  ScaleValues=1  scaleValueFracLength=14  stageInFracLength=15  stageOutFracLength=15
  Y_RMS2 : dsparch4/Digital Filter  DialogController=dspDDGCreate  DialogControllerArgs=DataTag137  TypePopup=IIR (poles & zeros)  IIRFiltStruct=Direct form II transposed  AllPoleFiltStruct=Direct form  FIRFiltStruct=Direct form  CoeffSource=Specify via dialog  NumCoeffs=[1 2]  DenCoeffs=[1 0.1]  BiQuadCoeffs=[1 0.3 0.4 1 0.1 0.2]  LatticeCoeffs=[0.2 0.4]  denIgnore=on  FiltPerSampPopup=One filter per frame  IC=0  ICnum=0  ICden=0  roundingMode=Floor  overflowMode=off  ScaleValues=1  scaleValueFracLength=14  stageInFracLength=15  stageOutFracLength=15
  Y_RMS_1 : cdsEpicsOut/Subsystem
  Y_RMS_2 : cdsEpicsOut/Subsystem
  Z : dsparch4/Digital Filter  DialogController=dspDDGCreate  DialogControllerArgs=DataTag138  TypePopup=IIR (poles & zeros)  IIRFiltStruct=Direct form II transposed  AllPoleFiltStruct=Direct form  FIRFiltStruct=Direct form  CoeffSource=Specify via dialog  NumCoeffs=[1 2]  DenCoeffs=[1 0.1]  BiQuadCoeffs=[1 0.3 0.4 1 0.1 0.2]  LatticeCoeffs=[0.2 0.4]  denIgnore=on  FiltPerSampPopup=One filter per frame  IC=0  ICnum=0  ICden=0  roundingMode=Floor  overflowMode=off  ScaleValues=1  scaleValueFracLength=14  stageInFracLength=15  stageOutFracLength=15
  Z_RMS : dsparch4/Digital Filter  DialogController=dspDDGCreate  DialogControllerArgs=DataTag139  TypePopup=IIR (poles & zeros)  IIRFiltStruct=Direct form II transposed  AllPoleFiltStruct=Direct form  FIRFiltStruct=Direct form  CoeffSource=Specify via dialog  NumCoeffs=[1 2]  DenCoeffs=[1 0.1]  BiQuadCoeffs=[1 0.3 0.4 1 0.1 0.2]  LatticeCoeffs=[0.2 0.4]  denIgnore=on  FiltPerSampPopup=One filter per frame  IC=0  ICnum=0  ICden=0  roundingMode=Floor  overflowMode=off  ScaleValues=1  scaleValueFracLength=14  stageInFracLength=15  stageOutFracLength=15
  Z_RMS2 : dsparch4/Digital Filter  DialogController=dspDDGCreate  DialogControllerArgs=DataTag140  TypePopup=IIR (poles & zeros)  IIRFiltStruct=Direct form II transposed  AllPoleFiltStruct=Direct form  FIRFiltStruct=Direct form  CoeffSource=Specify via dialog  NumCoeffs=[1 2]  DenCoeffs=[1 0.1]  BiQuadCoeffs=[1 0.3 0.4 1 0.1 0.2]  LatticeCoeffs=[0.2 0.4]  denIgnore=on  FiltPerSampPopup=One filter per frame  IC=0  ICnum=0  ICden=0  roundingMode=Floor  overflowMode=off  ScaleValues=1  scaleValueFracLength=14  stageInFracLength=15  stageOutFracLength=15
  Z_RMS_1 : cdsEpicsOut/Subsystem
  Z_RMS_2 : cdsEpicsOut/Subsystem
  rms{1..6} (6 alike) : cdsRms/Subsystem
  OutX : Outport
  OutY : Outport  Port=2
  OutZ : Outport  Port=3
  OutRx : Outport  Port=4
  OutRy : Outport  Port=5
  OutRz : Outport  Port=6
  OutVp : Outport  Port=7
  OutHp : Outport  Port=8
  wires:
  H2_IN/1 -> SH2/1
  H3_IN/1 -> SH3/1
  H4_IN/1 -> SH4/1
  MTRX/1 -> X/1, X_RMS2/1, X_RMS/1
  MTRX/2 -> Y/1, Y_RMS2/1, Y_RMS/1
  MTRX/3 -> Z/1, Z_RMS/1, Z_RMS2/1
  MTRX/6 -> RZ/1
  MTRX/7 -> VP/1
  MTRX/8 -> HP/1
  X/1 -> SW/1
  Y/1 -> SW/2
  Z/1 -> SW/3
  RX/1 -> SW/4
  RY/1 -> SW/5
  RZ/1 -> SW/6
  VP/1 -> SW/7
  HP/1 -> SW/8
  MTRX/4 -> RX/1
  MTRX/5 -> RY/1
  SW/1 -> OutX/1
  SW/2 -> OutY/1
  SW/3 -> OutZ/1
  SW/4 -> OutRx/1
  SW/5 -> OutRy/1
  SW/6 -> OutRz/1
  SW/7 -> OutVp/1
  SW/8 -> OutHp/1
  V1/1 -> MTRX/1
  V2/1 -> MTRX/2
  V3/1 -> MTRX/3
  V4/1 -> MTRX/4
  H1/1 -> MTRX/5
  H2/1 -> MTRX/6
  H3/1 -> MTRX/7
  H4/1 -> MTRX/8
  H1_IN/1 -> SH1/1
  V4_IN/1 -> SV4/1
  V3_IN/1 -> SV3/1
  V2_IN/1 -> SV2/1
  V1_IN/1 -> SV1/1
  SV1/1 -> Sum/1
  SV2/1 -> Sum1/1
  SV3/1 -> Sum2/1
  SV4/1 -> Sum3/1
  SH1/1 -> Sum4/1
  SH2/1 -> Sum5/1
  SH3/1 -> Sum6/1
  SH4/1 -> Sum7/1
  TV1/1 -> Sum/2
  TV2/1 -> Sum1/2
  TV3/1 -> Sum2/2
  TV4/1 -> Sum3/2
  TH1/1 -> Sum4/2
  TH2/1 -> Sum5/2
  TH3/1 -> Sum6/2
  TH4/1 -> Sum7/2
  Sum3/1 -> V4/1
  Sum4/1 -> H1/1
  Sum5/1 -> H2/1
  Sum6/1 -> H3/1
  Sum7/1 -> H4/1
  Sum/1 -> V1/1
  Sum1/1 -> V2/1
  Sum2/1 -> V3/1
  X_RMS_1/1 -> Terminator/1
  X_RMS_2/1 -> Terminator1/1
  Y_RMS_2/1 -> Terminator3/1
  Y_RMS_1/1 -> Terminator2/1
  Z_RMS_1/1 -> Terminator4/1
  Z_RMS_2/1 -> Terminator5/1
  X_RMS2/1 -> rms2/1
  X_RMS/1 -> rms1/1
  rms1/1 -> X_RMS_1/1
  rms2/1 -> X_RMS_2/1
  Y_RMS2/1 -> rms4/1
  Y_RMS/1 -> rms3/1
  rms3/1 -> Y_RMS_1/1
  rms4/1 -> Y_RMS_2/1
  Z_RMS2/1 -> rms6/1
  rms6/1 -> Z_RMS_2/1
  Z_RMS/1 -> rms5/1
  rms5/1 -> Z_RMS_1/1

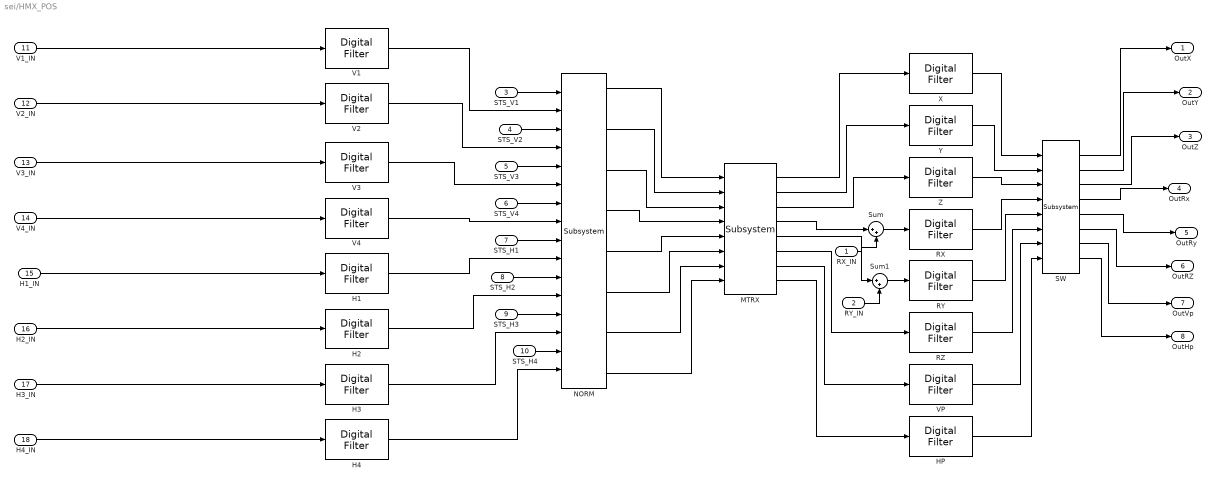
== system sei/HMX_POS ==
  RX_IN : Inport  Port=1  LatchInput=off
  RY_IN : Inport  Port=2  LatchInput=off
  STS_V1 : Inport  Port=3  LatchInput=off
  STS_V2 : Inport  Port=4  LatchInput=off
  STS_V3 : Inport  Port=5  LatchInput=off
  STS_V4 : Inport  Port=6  LatchInput=off
  STS_H1 : Inport  Port=7  LatchInput=off
  STS_H2 : Inport  Port=8  LatchInput=off
  STS_H3 : Inport  Port=9  LatchInput=off
  STS_H4 : Inport  Port=10  LatchInput=off
  V1_IN : Inport  Port=11  LatchInput=off
  V2_IN : Inport  Port=12  LatchInput=off
  V3_IN : Inport  Port=13  LatchInput=off
  V4_IN : Inport  Port=14  LatchInput=off
  H1_IN : Inport  Port=15  LatchInput=off
  H2_IN : Inport  Port=16  LatchInput=off
  H3_IN : Inport  Port=17  LatchInput=off
  H4_IN : Inport  Port=18  LatchInput=off
  H1 : dsparch4/Digital Filter  DialogController=dspDDGCreate  DialogControllerArgs=DataTag141  TypePopup=IIR (poles & zeros)  IIRFiltStruct=Direct form II transposed  AllPoleFiltStruct=Direct form  FIRFiltStruct=Direct form  CoeffSource=Specify via dialog  NumCoeffs=[1 2]  DenCoeffs=[1 0.1]  BiQuadCoeffs=[1 0.3 0.4 1 0.1 0.2]  LatticeCoeffs=[0.2 0.4]  denIgnore=on  FiltPerSampPopup=One filter per frame  IC=0  ICnum=0  ICden=0  roundingMode=Floor  overflowMode=off  ScaleValues=1  scaleValueFracLength=14  stageInFracLength=15  stageOutFracLength=15
  H2 : dsparch4/Digital Filter  DialogController=dspDDGCreate  DialogControllerArgs=DataTag142  TypePopup=IIR (poles & zeros)  IIRFiltStruct=Direct form II transposed  AllPoleFiltStruct=Direct form  FIRFiltStruct=Direct form  CoeffSource=Specify via dialog  NumCoeffs=[1 2]  DenCoeffs=[1 0.1]  BiQuadCoeffs=[1 0.3 0.4 1 0.1 0.2]  LatticeCoeffs=[0.2 0.4]  denIgnore=on  FiltPerSampPopup=One filter per frame  IC=0  ICnum=0  ICden=0  roundingMode=Floor  overflowMode=off  ScaleValues=1  scaleValueFracLength=14  stageInFracLength=15  stageOutFracLength=15
  H3 : dsparch4/Digital Filter  DialogController=dspDDGCreate  DialogControllerArgs=DataTag143  TypePopup=IIR (poles & zeros)  IIRFiltStruct=Direct form II transposed  AllPoleFiltStruct=Direct form  FIRFiltStruct=Direct form  CoeffSource=Specify via dialog  NumCoeffs=[1 2]  DenCoeffs=[1 0.1]  BiQuadCoeffs=[1 0.3 0.4 1 0.1 0.2]  LatticeCoeffs=[0.2 0.4]  denIgnore=on  FiltPerSampPopup=One filter per frame  IC=0  ICnum=0  ICden=0  roundingMode=Floor  overflowMode=off  ScaleValues=1  scaleValueFracLength=14  stageInFracLength=15  stageOutFracLength=15
  H4 : dsparch4/Digital Filter  DialogController=dspDDGCreate  DialogControllerArgs=DataTag144  TypePopup=IIR (poles & zeros)  IIRFiltStruct=Direct form II transposed  AllPoleFiltStruct=Direct form  FIRFiltStruct=Direct form  CoeffSource=Specify via dialog  NumCoeffs=[1 2]  DenCoeffs=[1 0.1]  BiQuadCoeffs=[1 0.3 0.4 1 0.1 0.2]  LatticeCoeffs=[0.2 0.4]  denIgnore=on  FiltPerSampPopup=One filter per frame  IC=0  ICnum=0  ICden=0  roundingMode=Floor  overflowMode=off  ScaleValues=1  scaleValueFracLength=14  stageInFracLength=15  stageOutFracLength=15
  HP : dsparch4/Digital Filter  DialogController=dspDDGCreate  DialogControllerArgs=DataTag145  TypePopup=IIR (poles & zeros)  IIRFiltStruct=Direct form II transposed  AllPoleFiltStruct=Direct form  FIRFiltStruct=Direct form  CoeffSource=Specify via dialog  NumCoeffs=[1 2]  DenCoeffs=[1 0.1]  BiQuadCoeffs=[1 0.3 0.4 1 0.1 0.2]  LatticeCoeffs=[0.2 0.4]  denIgnore=on  FiltPerSampPopup=One filter per frame  IC=0  ICnum=0  ICden=0  roundingMode=Floor  overflowMode=off  ScaleValues=1  scaleValueFracLength=14  stageInFracLength=15  stageOutFracLength=15
  MTRX : Matrix8x/Subsystem
  NORM : cdsSubtract8/Subsystem
  RX : dsparch4/Digital Filter  DialogController=dspDDGCreate  DialogControllerArgs=DataTag146  TypePopup=IIR (poles & zeros)  IIRFiltStruct=Direct form II transposed  AllPoleFiltStruct=Direct form  FIRFiltStruct=Direct form  CoeffSource=Specify via dialog  NumCoeffs=[1 2]  DenCoeffs=[1 0.1]  BiQuadCoeffs=[1 0.3 0.4 1 0.1 0.2]  LatticeCoeffs=[0.2 0.4]  denIgnore=on  FiltPerSampPopup=One filter per frame  IC=0  ICnum=0  ICden=0  roundingMode=Floor  overflowMode=off  ScaleValues=1  scaleValueFracLength=14  stageInFracLength=15  stageOutFracLength=15
  RY : dsparch4/Digital Filter  DialogController=dspDDGCreate  DialogControllerArgs=DataTag147  TypePopup=IIR (poles & zeros)  IIRFiltStruct=Direct form II transposed  AllPoleFiltStruct=Direct form  FIRFiltStruct=Direct form  CoeffSource=Specify via dialog  NumCoeffs=[1 2]  DenCoeffs=[1 0.1]  BiQuadCoeffs=[1 0.3 0.4 1 0.1 0.2]  LatticeCoeffs=[0.2 0.4]  denIgnore=on  FiltPerSampPopup=One filter per frame  IC=0  ICnum=0  ICden=0  roundingMode=Floor  overflowMode=off  ScaleValues=1  scaleValueFracLength=14  stageInFracLength=15  stageOutFracLength=15
  RZ : dsparch4/Digital Filter  DialogController=dspDDGCreate  DialogControllerArgs=DataTag148  TypePopup=IIR (poles & zeros)  IIRFiltStruct=Direct form II transposed  AllPoleFiltStruct=Direct form  FIRFiltStruct=Direct form  CoeffSource=Specify via dialog  NumCoeffs=[1 2]  DenCoeffs=[1 0.1]  BiQuadCoeffs=[1 0.3 0.4 1 0.1 0.2]  LatticeCoeffs=[0.2 0.4]  denIgnore=on  FiltPerSampPopup=One filter per frame  IC=0  ICnum=0  ICden=0  roundingMode=Floor  overflowMode=off  ScaleValues=1  scaleValueFracLength=14  stageInFracLength=15  stageOutFracLength=15
  SW : cdsSwitch/Subsystem
  Sum : Sum  Inputs=|++
  Sum1 : Sum  Inputs=|++
  V1 : dsparch4/Digital Filter  DialogController=dspDDGCreate  DialogControllerArgs=DataTag149  TypePopup=IIR (poles & zeros)  IIRFiltStruct=Direct form II transposed  AllPoleFiltStruct=Direct form  FIRFiltStruct=Direct form  CoeffSource=Specify via dialog  NumCoeffs=[1 2]  DenCoeffs=[1 0.1]  BiQuadCoeffs=[1 0.3 0.4 1 0.1 0.2]  LatticeCoeffs=[0.2 0.4]  denIgnore=on  FiltPerSampPopup=One filter per frame  IC=0  ICnum=0  ICden=0  roundingMode=Floor  overflowMode=off  ScaleValues=1  scaleValueFracLength=14  stageInFracLength=15  stageOutFracLength=15
  V2 : dsparch4/Digital Filter  DialogController=dspDDGCreate  DialogControllerArgs=DataTag150  TypePopup=IIR (poles & zeros)  IIRFiltStruct=Direct form II transposed  AllPoleFiltStruct=Direct form  FIRFiltStruct=Direct form  CoeffSource=Specify via dialog  NumCoeffs=[1 2]  DenCoeffs=[1 0.1]  BiQuadCoeffs=[1 0.3 0.4 1 0.1 0.2]  LatticeCoeffs=[0.2 0.4]  denIgnore=on  FiltPerSampPopup=One filter per frame  IC=0  ICnum=0  ICden=0  roundingMode=Floor  overflowMode=off  ScaleValues=1  scaleValueFracLength=14  stageInFracLength=15  stageOutFracLength=15
  V3 : dsparch4/Digital Filter  DialogController=dspDDGCreate  DialogControllerArgs=DataTag151  TypePopup=IIR (poles & zeros)  IIRFiltStruct=Direct form II transposed  AllPoleFiltStruct=Direct form  FIRFiltStruct=Direct form  CoeffSource=Specify via dialog  NumCoeffs=[1 2]  DenCoeffs=[1 0.1]  BiQuadCoeffs=[1 0.3 0.4 1 0.1 0.2]  LatticeCoeffs=[0.2 0.4]  denIgnore=on  FiltPerSampPopup=One filter per frame  IC=0  ICnum=0  ICden=0  roundingMode=Floor  overflowMode=off  ScaleValues=1  scaleValueFracLength=14  stageInFracLength=15  stageOutFracLength=15
  V4 : dsparch4/Digital Filter  DialogController=dspDDGCreate  DialogControllerArgs=DataTag152  TypePopup=IIR (poles & zeros)  IIRFiltStruct=Direct form II transposed  AllPoleFiltStruct=Direct form  FIRFiltStruct=Direct form  CoeffSource=Specify via dialog  NumCoeffs=[1 2]  DenCoeffs=[1 0.1]  BiQuadCoeffs=[1 0.3 0.4 1 0.1 0.2]  LatticeCoeffs=[0.2 0.4]  denIgnore=on  FiltPerSampPopup=One filter per frame  IC=0  ICnum=0  ICden=0  roundingMode=Floor  overflowMode=off  ScaleValues=1  scaleValueFracLength=14  stageInFracLength=15  stageOutFracLength=15
  VP : dsparch4/Digital Filter  DialogController=dspDDGCreate  DialogControllerArgs=DataTag153  TypePopup=IIR (poles & zeros)  IIRFiltStruct=Direct form II transposed  AllPoleFiltStruct=Direct form  FIRFiltStruct=Direct form  CoeffSource=Specify via dialog  NumCoeffs=[1 2]  DenCoeffs=[1 0.1]  BiQuadCoeffs=[1 0.3 0.4 1 0.1 0.2]  LatticeCoeffs=[0.2 0.4]  denIgnore=on  FiltPerSampPopup=One filter per frame  IC=0  ICnum=0  ICden=0  roundingMode=Floor  overflowMode=off  ScaleValues=1  scaleValueFracLength=14  stageInFracLength=15  stageOutFracLength=15
  X : dsparch4/Digital Filter  DialogController=dspDDGCreate  DialogControllerArgs=DataTag154  TypePopup=IIR (poles & zeros)  IIRFiltStruct=Direct form II transposed  AllPoleFiltStruct=Direct form  FIRFiltStruct=Direct form  CoeffSource=Specify via dialog  NumCoeffs=[1 2]  DenCoeffs=[1 0.1]  BiQuadCoeffs=[1 0.3 0.4 1 0.1 0.2]  LatticeCoeffs=[0.2 0.4]  denIgnore=on  FiltPerSampPopup=One filter per frame  IC=0  ICnum=0  ICden=0  roundingMode=Floor  overflowMode=off  ScaleValues=1  scaleValueFracLength=14  stageInFracLength=15  stageOutFracLength=15
  Y : dsparch4/Digital Filter  DialogController=dspDDGCreate  DialogControllerArgs=DataTag155  TypePopup=IIR (poles & zeros)  IIRFiltStruct=Direct form II transposed  AllPoleFiltStruct=Direct form  FIRFiltStruct=Direct form  CoeffSource=Specify via dialog  NumCoeffs=[1 2]  DenCoeffs=[1 0.1]  BiQuadCoeffs=[1 0.3 0.4 1 0.1 0.2]  LatticeCoeffs=[0.2 0.4]  denIgnore=on  FiltPerSampPopup=One filter per frame  IC=0  ICnum=0  ICden=0  roundingMode=Floor  overflowMode=off  ScaleValues=1  scaleValueFracLength=14  stageInFracLength=15  stageOutFracLength=15
  Z : dsparch4/Digital Filter  DialogController=dspDDGCreate  DialogControllerArgs=DataTag156  TypePopup=IIR (poles & zeros)  IIRFiltStruct=Direct form II transposed  AllPoleFiltStruct=Direct form  FIRFiltStruct=Direct form  CoeffSource=Specify via dialog  NumCoeffs=[1 2]  DenCoeffs=[1 0.1]  BiQuadCoeffs=[1 0.3 0.4 1 0.1 0.2]  LatticeCoeffs=[0.2 0.4]  denIgnore=on  FiltPerSampPopup=One filter per frame  IC=0  ICnum=0  ICden=0  roundingMode=Floor  overflowMode=off  ScaleValues=1  scaleValueFracLength=14  stageInFracLength=15  stageOutFracLength=15
  OutX : Outport
  OutY : Outport  Port=2
  OutZ : Outport  Port=3
  OutRx : Outport  Port=4
  OutRy : Outport  Port=5
  OutRZ : Outport  Port=6
  OutVp : Outport  Port=7
  OutHp : Outport  Port=8
  wires:
  V1_IN/1 -> V1/1
  V2_IN/1 -> V2/1
  V3_IN/1 -> V3/1
  V4_IN/1 -> V4/1
  H1_IN/1 -> H1/1
  H2_IN/1 -> H2/1
  H3_IN/1 -> H3/1
  H4_IN/1 -> H4/1
  V1/1 -> NORM/2
  V2/1 -> NORM/4
  V3/1 -> NORM/6
  V4/1 -> NORM/8
  H1/1 -> NORM/10
  H2/1 -> NORM/12
  H3/1 -> NORM/14
  H4/1 -> NORM/16
  STS_V1/1 -> NORM/1
  STS_V2/1 -> NORM/3
  STS_V3/1 -> NORM/5
  STS_V4/1 -> NORM/7
  STS_H1/1 -> NORM/9
  STS_H2/1 -> NORM/11
  STS_H3/1 -> NORM/13
  STS_H4/1 -> NORM/15
  MTRX/1 -> X/1
  MTRX/2 -> Y/1
  MTRX/3 -> Z/1
  MTRX/6 -> RZ/1
  MTRX/7 -> VP/1
  MTRX/8 -> HP/1
  Sum1/1 -> RY/1
  Sum/1 -> RX/1
  MTRX/4 -> Sum/1
  MTRX/5 -> Sum1/1
  X/1 -> SW/1
  Y/1 -> SW/2
  Z/1 -> SW/3
  RX/1 -> SW/4
  RY/1 -> SW/5
  RZ/1 -> SW/6
  VP/1 -> SW/7
  HP/1 -> SW/8
  RX_IN/1 -> Sum/2
  RY_IN/1 -> Sum1/2
  NORM/1 -> MTRX/1
  NORM/2 -> MTRX/2
  NORM/3 -> MTRX/3
  NORM/4 -> MTRX/4
  NORM/5 -> MTRX/5
  NORM/6 -> MTRX/6
  NORM/7 -> MTRX/7
  NORM/8 -> MTRX/8
  SW/1 -> OutX/1
  SW/2 -> OutY/1
  SW/3 -> OutZ/1
  SW/4 -> OutRx/1
  SW/5 -> OutRy/1
  SW/6 -> OutRZ/1
  SW/7 -> OutVp/1
  SW/8 -> OutHp/1
